simulink model "mstf_withEV"  (R2021a)
settings: Solver=VariableStepAuto  StartTime=0.0  StopTime=3  RelTol=1e-3
undefined symbols (not defined in the file or in its folder): Ion, Lithium
libraries: spsCurrentMeasurementLib x25, spsVoltageMeasurementLib x19, spsSeriesRLCBranchLib x11, spsGroundLib x6, powerlib_extras x5, dspsigops x3, spsPower3phInstantaneousLib x3, eeTotalHarmonicDistorsion x3, spsIGBTDiodeLib x2, spsUniversalBridgeLib x2, spsBatteryLib x1, spsParallelRLCBranchLib x1
settings Model: Creator=Dell  LastModifiedBy=Dell
settings SolverCC: ZeroCrossControl=DisableAll

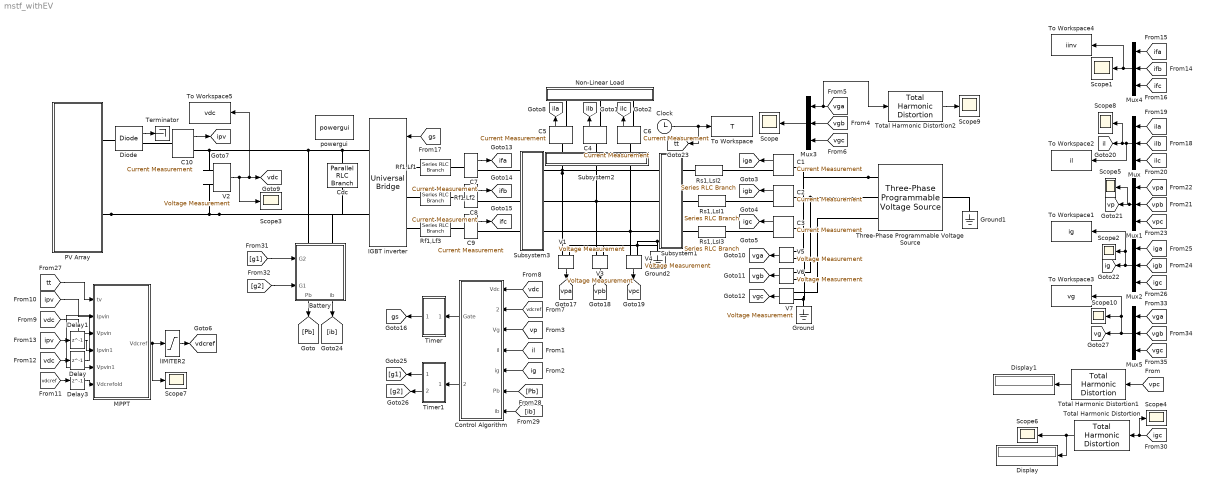
== system mstf_withEV ==
  Battery : Subsystem
      settings: PortSchema="{\"entries\":[{\"content\":{\"sides\":[{\"content\":{\"connectorIds\":[\"LConn1\",\"LConn2\"]},\"type\":\"ConnectorPlacement.EquallySpacedRectSide\",\"uuid\":\"3f024d4f-4944-46f1-a681-19b9b6f5c2e3\"},{\"content\":{\"connectorIds\":[\"Out1\",\"Out2\"],\"side\":\"RIGHT\"},\"type\":\"ConnectorPlacement.EquallySpacedRectSide\",\"uuid\":\"ba9189b8-b241-4d0f-92c2-ffae32477602\"},{\"content\":{\"connectorIds\":[\"In1\",\"In2\"],\"side\":\"TOP\"},\"type\":\"ConnectorPlacement.EquallySpacedRectSide\",\"uuid\":\"2b5a68b6-4f88-4313-be0a-70c6e84ce948\"}]},\"type\":\"ConnectorPlacement.EquallySpacedConnector\",\"uuid\":\"57f7ac83-2601-4f06-be16-46ca99d36a1f\"}],\"packageUris\":[\"http://schema.mathworks.com/mf0/Connector/R2020b\"],\"version\":\"1.0\"}"
  C{1..10} (10 alike) : spsCurrentMeasurementLib/Current Measurement  PhasorSimulation=off  OutputType=Complex  PSBequivalent=0
  Cdc : spsParallelRLCBranchLib/Parallel RLC Branch  LConnTagsString=a  RConnTagsString=__new0  BranchType=C  Resistance=10  Inductance=1.0  SetiL0=off  InitialCurrent=0  Capacitance=800e-6  Setx0=on  InitialVoltage=810  Measurements=None
  Clock : Clock
  Control Algorithm : Subsystem
  Delay : Delay  DelayLength=1  InitialCondition=0  InputProcessing=Columns as channels (frame based)
  Delay1 : Delay  DelayLength=1  InitialCondition=0  InputProcessing=Columns as channels (frame based)
  Delay3 : Delay  DelayLength=1  InitialCondition=810  InputProcessing=Columns as channels (frame based)
  Diode : spsDiodeLib/Diode  Ron=0.001  Lon=0  Vf=0.8  IC=0  UseSnubber=off  Rs=500  Cs=250e-9  Measurements=on
  Display : Display
  Display1 : Display
  Ground : spsGroundLib/Ground  LConnTagsString=a
  Ground1 : spsGroundLib/Ground  LConnTagsString=a
  Ground2 : spsGroundLib/Ground  LConnTagsString=a
  IGBT inverter : spsUniversalBridgeLib/Universal Bridge  Arms=3  SnubberResistance=1e5  SnubberCapacitance=inf  Device=IGBT / Diodes  Ron=1e-3  Lon=0  ForwardVoltages="[  0  0  ]"  ForwardVoltage=0  GTOparameters=[ 10e-6 , 20e-6 ]  IGBTparameters=[ 1e-6 , 2e-6 ]  Measurements=Device voltages  Measurements_2=None  converterType=Rectifier
  MPPT : MATLAB Function  TreatAsAtomicUnit=on
  Mux{,1..5} (6 alike) : Mux  Inputs=3
  Non-Linear Load : Subsystem
  PV Array : Subsystem
  Rf1,Lf1 : spsSeriesRLCBranchLib/Series RLC Branch  LConnTagsString=__new0  RConnTagsString=__new0  BranchType=RL  Resistance=.01  Inductance=10e-3  SetiL0=off  InitialCurrent=0  Capacitance=1e-6  Setx0=off  InitialVoltage=0  Measurements=None
  Rf1,Lf2 : spsSeriesRLCBranchLib/Series RLC Branch  LConnTagsString=__new0  RConnTagsString=__new0  BranchType=RL  Resistance=.01  Inductance=10e-3  SetiL0=off  InitialCurrent=0  Capacitance=1e-6  Setx0=off  InitialVoltage=0  Measurements=None
  Rf1,Lf3 : spsSeriesRLCBranchLib/Series RLC Branch  LConnTagsString=__new0  RConnTagsString=__new0  BranchType=RL  Resistance=.01  Inductance=10e-3  SetiL0=off  InitialCurrent=0  Capacitance=1e-6  Setx0=off  InitialVoltage=0  Measurements=None
  Rs1,LsI1 : spsSeriesRLCBranchLib/Series RLC Branch  LConnTagsString=__new0  RConnTagsString=__new0  BranchType=RL  Resistance=.1  Inductance=0.5e-3  SetiL0=off  InitialCurrent=0  Capacitance=1e-6  Setx0=off  InitialVoltage=0  Measurements=None
  Rs1,LsI2 : spsSeriesRLCBranchLib/Series RLC Branch  LConnTagsString=__new0  RConnTagsString=__new0  BranchType=RL  Resistance=.1  Inductance=0.5e-3  SetiL0=off  InitialCurrent=0  Capacitance=1e-6  Setx0=off  InitialVoltage=0  Measurements=None
  Rs1,LsI3 : spsSeriesRLCBranchLib/Series RLC Branch  LConnTagsString=__new0  RConnTagsString=__new0  BranchType=RL  Resistance=.1  Inductance=0.5e-3  SetiL0=off  InitialCurrent=0  Capacitance=1e-6  Setx0=off  InitialVoltage=0  Measurements=None
  Scope{,1..10} (11 alike) : Scope
  Subsystem1 : Subsystem
  Subsystem2 : Subsystem
  Subsystem3 : Subsystem
  Terminator : Terminator
  Three-Phase Programmable Voltage Source : spsThreePhaseProgrammableVoltageSourceLib/Three-Phase Programmable Voltage Source  PositiveSequence="[400  0 50]"  VariationEntity=None  VariationType=Table of time-amplitude pairs  VariationTypeAlt=Step  VariationStep=0.5  VariationRate=10  VariationMagnitude=0.3  VariationFrequency=2  VariationTiming=[1 2]  VariationPhaseA=off  Amplitudes=[1 0.8 1.2 1.0]  TimeValues=[0 0.1 0.15 0.2]  HarmonicGeneration=on  HarmonicA=[3 0.02 -25 0]  HarmonicB=[5 0.03 35 2]  Timing="[0.05  3]"  BusType=swing  Pref=0  Qref=0  Qmin=-inf  Qmax=inf
  Timer : Subsystem
  Timer1 : Subsystem
  To Workspace : ToWorkspace  VariableName=T  SampleTime=-1
      settings: MaxDataPoints=614863
  To Workspace1 : ToWorkspace  VariableName=ig  SampleTime=-1
      settings: MaxDataPoints=614863
  To Workspace2 : ToWorkspace  VariableName=il  SampleTime=-1
      settings: MaxDataPoints=614863
  To Workspace3 : ToWorkspace  VariableName=vg  SampleTime=-1
      settings: MaxDataPoints=614863
  To Workspace4 : ToWorkspace  VariableName=iinv  SampleTime=-1
      settings: MaxDataPoints=614863
  To Workspace5 : ToWorkspace  VariableName=vdc  SampleTime=-1
      settings: MaxDataPoints=614863
  Total Harmonic Distortion : eeTotalHarmonicDistorsion/Total Harmonic Distortion  f=50  Ts=-1
      settings: SourceProductBaseCode=PS
  Total Harmonic Distortion1 : eeTotalHarmonicDistorsion/Total Harmonic Distortion  f=50  Ts=-1
      settings: SourceProductBaseCode=PS
  Total Harmonic Distortion2 : eeTotalHarmonicDistorsion/Total Harmonic Distortion  f=50  Ts=-1
      settings: SourceProductBaseCode=PS
  V{1..7} (7 alike) : spsVoltageMeasurementLib/Voltage Measurement  PhasorSimulation=off  OutputType=Complex  PSBequivalent=0
  lIMITER2 : Saturate  UpperLimit=820  LowerLimit=630
  powergui : spspowerguiLib/powergui  Priority=1  SimulationMode=Discrete  SampleTime=5e-6  frequency=60  Iterations=50  frequencyindice=50  Pbase=100e6  ErrMax=1e-4  UnitsV=kV  UnitsW=MW  buscounter=0  FunctionMessages=off  echomessages=off  EnableUseOfTLC=off  CurrentSourceSwitches=off  DisableSnubberDevices=off  DisableRonSwitches=off  DisableVfSwitches=off  DisplayEquations=off  AutomaticDiscreteSolvers=off  SolverType=Tustin  Interpol=off  ExternalGateDelay=off  methode=off  Ts=0  x0status=blocks  SPID=off  SwTol=0  HookPort=off  NonlinearTolerance=1e-4  nMaxIteration=100  ContinueOnMaxIteration=off  RestoreLinks=warning  ResistiveCurrentMeasurement=off  Frange=[0:2:500]  Ylog=off  Xlog=on  ShowGrid=off  save=off  variable=ZData  structure=sourcect6  ZoomFFT=off  StartTime=1.81  cycles=3  DisplayStyle=3  fundamental=50  FreqAxis=on  MaxFrequency=1000  frequencyindicesteady=1  RmsSteady=1  display=off
  tag scope: gs=global, ifa=global, ifb=global, ifc=global, ig=global, iga=global, igb=global, igc=global, il=global, ila=global, ilb=global, ilc=global, ipv=global, tt=global, vdc=global, vdcref=global, vg=global, vga=global, vgb=global, vgc=global, vp=global, vpa=global, vpb=global, vpc=global
  wires:
  C3/1 -> [igc]
  [iga] -> Mux2/1
  Mux5/1 -> Scope10/1, To Workspace3/1, [vg]
  [vgb] -> Mux5/2
  Battery/2(ib) -> [ib]
  V6/1 -> [vgb]
  lIMITER2/1 -> [vdcref]
  [vga] -> Mux5/1
  [ib] -> Control Algorithm/7(ib)
  Control Algorithm/2(gate2) -> Timer1/1(In1)
  Diode/1 -> Terminator/1
  [vdcref] -> Control Algorithm/2(Vdcref)
  [vgc] -> Mux5/3
  [Pb] -> Control Algorithm/6(Pb)
  [vga] -> Total Harmonic Distortion2/1, Mux3/1
  [igc] -> Scope4/1, Total Harmonic Distortion/1
  [vgc] -> Mux3/3
  Total Harmonic Distortion2/1 -> Scope9/1
  [ila] -> Mux/1
  [g1] -> Battery/1(G2)
  Battery/1(Pb) -> [Pb]
  [ig] -> Control Algorithm/5(ig)
  Mux1/1 -> Scope5/1, [vp]
  [vpc] -> Total Harmonic Distortion1/1
  [tt] -> MPPT/1(tv)
  Mux4/1 -> To Workspace4/1, Scope1/1
  Total Harmonic Distortion1/1 -> Display1/1
  [ifb] -> Mux4/2
  [vpc] -> Mux1/3
  V1/1 -> [vpa]
  Total Harmonic Distortion/1 -> Scope6/1, Display/1
  [vp] -> Control Algorithm/3(Vg)
  [igc] -> Mux2/3
  MPPT/1(Vdcref) -> Scope7/1, lIMITER2/1
  Mux3/1 -> Scope/1
  [vdcref] -> Delay3/1
  [ifc] -> Mux4/3
  [il] -> Control Algorithm/4(il)
  Mux2/1 -> To Workspace1/1, Scope2/1, [ig]
  V3/1 -> [vpb]
  V5/1 -> [vga]
  [igb] -> Mux2/2
  [vpb] -> Mux1/2
  Control Algorithm/1(Gate) -> Timer/1(In1)
  C5/1 -> [ila]
  V2/1 -> To Workspace5/1, [vdc], Scope3/1
  [vpa] -> Mux1/1
  Delay1/1 -> MPPT/4(Ipvin1)
  [ilb] -> Mux/2
  C2/1 -> [igb]
  [gs] -> IGBT inverter/1
  C4/1 -> [ilb]
  [g2] -> Battery/2(G1)
  C9/1 -> [ifc]
  Timer/1(Out1) -> [gs]
  C8/1 -> [ifb]
  Timer1/1(g1) -> [g1]
  Delay3/1 -> MPPT/6(Vdcrefold)
  C7/1 -> [ifa]
  V7/1 -> [vgc]
  Clock/1 -> [tt], To Workspace/1
  C10/1 -> [ipv]
  [ipv] -> Delay1/1
  [vdc] -> MPPT/3(Vpvin)
  Delay/1 -> MPPT/5(Vpvin1)
  C1/1 -> [iga]
  [ipv] -> MPPT/2(Ipvin)
  [ifa] -> Mux4/1
  [vdc] -> Control Algorithm/1(Vdc)
  Mux/1 -> To Workspace2/1, [il], Scope8/1
  V4/1 -> [vpc]
  Timer1/2(g2) -> [g2]
  [ilc] -> Mux/3
  C6/1 -> [ilc]
  [vgb] -> Mux3/2
  [vdc] -> Delay/1
  connections:
  V6/LConn2 -- Ground/LConn1 -- V7/LConn2 -- V5/LConn2
  V7/LConn1 -- C3/LConn1 -- Three-Phase Programmable Voltage Source/RConn3
  V2/LConn1 -- IGBT inverter/RConn1 -- Cdc/LConn1 -- Battery/LConn1 -- C10/RConn1
  Subsystem2/LConn3 -- V4/LConn1 -- Subsystem3/RConn3 -- Subsystem1/RConn3
  Subsystem1/RConn2 -- V3/LConn1 -- Subsystem2/LConn2 -- Subsystem3/RConn2
  Subsystem2/LConn1 -- Subsystem1/RConn1 -- Subsystem3/RConn1 -- V1/LConn1
  Three-Phase Programmable Voltage Source/RConn1 -- C1/LConn1 -- V5/LConn1
  Ground2/LConn1 -- V3/LConn2 -- V1/LConn2 -- V4/LConn2
  PV Array/LConn2 -- IGBT inverter/RConn2 -- Cdc/RConn1 -- Battery/LConn2 -- V2/LConn2
  Three-Phase Programmable Voltage Source/RConn2 -- C2/LConn1 -- V6/LConn1
  Rs1,LsI3/RConn1 -- C3/RConn1
  Subsystem2/RConn3 -- C6/LConn1
  C8/LConn1 -- Rf1,Lf2/RConn1
  C4/LConn1 -- Subsystem2/RConn2
  Subsystem3/LConn1 -- C7/RConn1
  IGBT inverter/LConn1 -- Rf1,Lf1/LConn1
  Diode/RConn1 -- C10/LConn1
  Rs1,LsI3/LConn1 -- Subsystem1/LConn3
  C9/LConn1 -- Rf1,Lf3/RConn1
  Non-Linear Load/LConn1 -- C5/RConn1
  C9/RConn1 -- Subsystem3/LConn3
  Non-Linear Load/LConn2 -- C4/RConn1
  C2/RConn1 -- Rs1,LsI1/RConn1
  PV Array/LConn1 -- Diode/LConn1
  Rf1,Lf2/LConn1 -- IGBT inverter/LConn2
  Rs1,LsI2/LConn1 -- Subsystem1/LConn1
  Non-Linear Load/LConn3 -- C6/RConn1
  Rs1,LsI2/RConn1 -- C1/RConn1
  Rf1,Lf3/LConn1 -- IGBT inverter/LConn3
  Ground1/LConn1 -- Three-Phase Programmable Voltage Source/LConn1
  Rf1,Lf1/RConn1 -- C7/LConn1
  C5/LConn1 -- Subsystem2/RConn1
  Rs1,LsI1/LConn1 -- Subsystem1/LConn2
  C8/RConn1 -- Subsystem3/LConn2

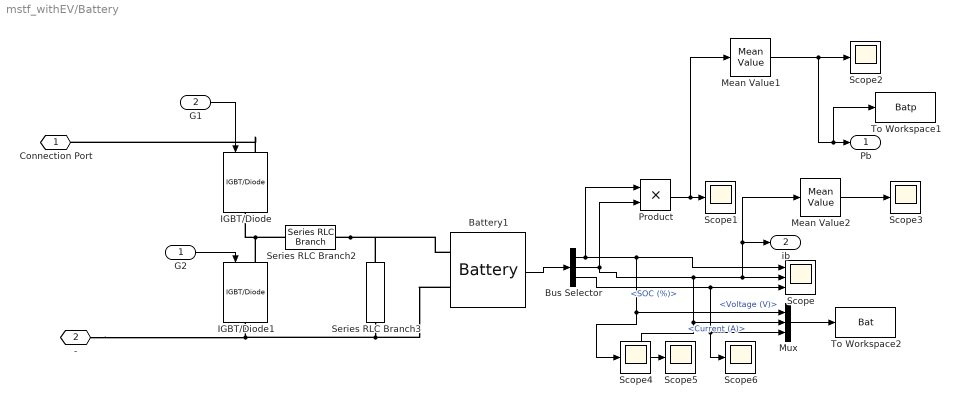
== system mstf_withEV/Battery ==
  G2 : Inport
  G1 : Inport  Port=2
  Battery1 : spsBatteryLib/Battery  BatType=Lithium-Ion  ShowTempParam=off  ThermalPreset=no  ShowAgeParam=off  NomV=300  NomQ=10  SOC=9  Batt_Tr=1  PresetModel=on  MaxQ=10  MinV=225  FullV=349.1961  Dis_rate=4.3478  R=0.3  Normal_OP=9.0435  expZone="[324.1158     0.4913043]"  current=[6.5 13 32.5]  Units=Time  Tci=20  NomT=20  T2=-30  MaxQ2=4.8  FullV2=7.1  Normal_OP2=5.655  expZone2="[6.58           1]"  Rca=0.6  ti=2000  Dp=0  Neq0=0  Tsim=1e6  Ta1=25  Qeol=5.4*0.9  Reol=0.013333*1.2  Char_age=[2.3478, 3]  Dis_age=[2.3478, 10]  N1=1500  N2=10500  N3=1000  N4=1400  Ta2=45  N5=950
  Bus Selector : BusSelector  OutputSignals=Voltage (V),Current (A),SOC (%)
  IGBT/Diode : spsIGBTDiodeLib/IGBT//Diode  Ron=1e-3  Rs=1e5  Cs=inf  Measurements=off
  IGBT/Diode1 : spsIGBTDiodeLib/IGBT//Diode  Ron=1e-3  Rs=1e5  Cs=inf  Measurements=off
  Mean Value1 : powerlib_extras/Measurements/Mean Value  Period=1/100
      settings: SourceProductBaseCode=PS
  Mean Value2 : powerlib_extras/Measurements/Mean Value  Period=1/100
      settings: SourceProductBaseCode=PS
  Mux : Mux  Inputs=3
  Product : Product
  Scope : Scope  NumInputPorts=3
  Scope{1..6} (6 alike) : Scope
  Series RLC Branch2 : spsSeriesRLCBranchLib/Series RLC Branch  LConnTagsString=__new0  RConnTagsString=__new0  BranchType=L  Resistance=1  Inductance=2e-3  SetiL0=off  InitialCurrent=0  Capacitance=1e-6  Setx0=off  InitialVoltage=0  Measurements=None
  Series RLC Branch3 : spsSeriesRLCBranchLib/Series RLC Branch  LConnTagsString=__new0  RConnTagsString=__new0  BranchType=C  Resistance=1  Inductance=1e-3  SetiL0=off  InitialCurrent=0  Capacitance=1000e-6  Setx0=off  InitialVoltage=0  Measurements=None
  To Workspace1 : ToWorkspace  VariableName=Batp  SampleTime=-1
      settings: MaxDataPoints=614863
  To Workspace2 : ToWorkspace  VariableName=Bat  SampleTime=-1
      settings: MaxDataPoints=614863
  Connection Port : PMIOPort  Side=Left
  - : PMIOPort  Port=2  Side=Left
  Pb : Outport
  ib : Outport  Port=2
  wires:
  Battery1/1 -> Bus Selector/1
  Bus Selector/1 -> Product/1, Scope/1, Mux/1, Scope4/1  "<Voltage (V)>"
  Bus Selector/2 -> Scope/2, ib/1, Mean Value2/1, Mux/2, Scope5/1, Product/2  "<Current (A)>"
  G1/1 -> IGBT/Diode/1
  G2/1 -> IGBT/Diode1/1
  Product/1 -> Mean Value1/1, Scope1/1
  Bus Selector/3 -> Scope/3, Mux/3, Scope6/1  "<SOC (%)>"
  Mean Value1/1 -> To Workspace1/1, Pb/1, Scope2/1
  Mean Value2/1 -> Scope3/1
  Mux/1 -> To Workspace2/1
  connections:
  Series RLC Branch2/RConn1 -- Battery1/LConn1 -- Series RLC Branch3/LConn1
  IGBT/Diode1/LConn1 -- Series RLC Branch2/LConn1 -- IGBT/Diode/RConn1
  Series RLC Branch3/RConn1 -- Battery1/LConn2 -- -/RConn1 -- IGBT/Diode1/RConn1
  IGBT/Diode/LConn1 -- Connection Port/RConn1

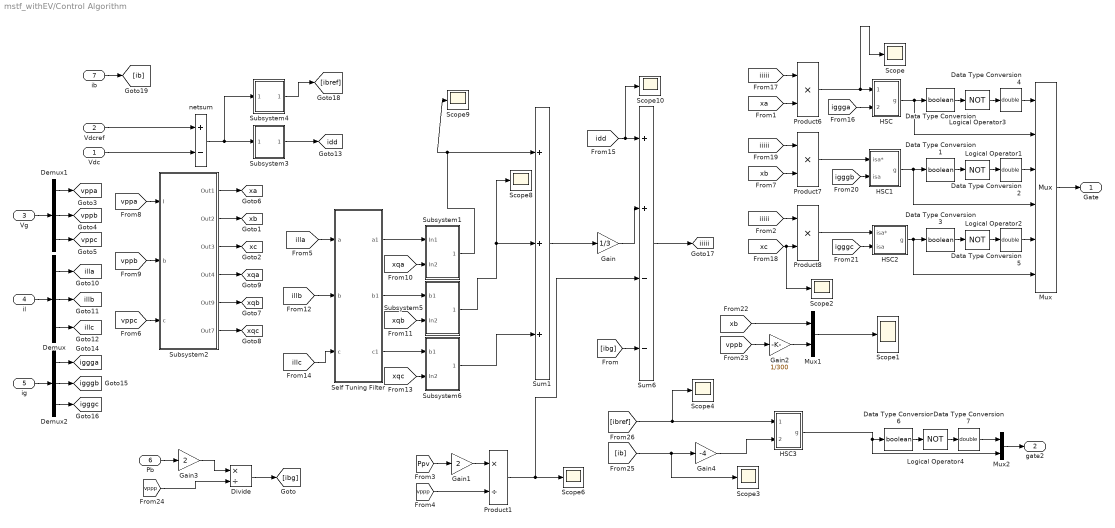
== system mstf_withEV/Control Algorithm ==
  Vdc : Inport
  Vdcref : Inport  Port=2
  Vg : Inport  Port=3
  il : Inport  Port=4
  ig : Inport  Port=5
  Pb : Inport  Port=6
  ib : Inport  Port=7
  Data Type Conversion{,1,3,6} (4 alike) : DataTypeConversion  OutDataTypeStr=boolean  SaturateOnIntegerOverflow=on  RndMeth=Zero
  Data Type Conversion{2,4..5,7} (4 alike) : DataTypeConversion  OutDataTypeStr=double  SaturateOnIntegerOverflow=on  RndMeth=Zero
  Demux : Demux  Outputs=3
  Demux1 : Demux  Outputs=3
  Demux2 : Demux  Outputs=3
  Divide : Product  Inputs=*/
  Gain : Gain  Gain=1/3
  Gain1 : Gain  Gain=2
  Gain2 : Gain  Gain=1/300
  Gain3 : Gain  Gain=2
  Gain4 : Gain  Gain=-4
  HSC : Subsystem  mask{h=.005}
      mask prompts: h "Hysteresis band (A)"
      mask help: Hysteresis Current Controller
      mask Display: plot(0,0,100,100,[45,45],[35,65],[55,55],[35,65],[45,65],[65,65],[35,55],[35,35])
  HSC1 : Subsystem  mask{h=.005}
      mask prompts: h "Hysteresis band (A)"
      mask help: Hysteresis Current Controller
      mask Display: plot(0,0,100,100,[45,45],[35,65],[55,55],[35,65],[45,65],[65,65],[35,55],[35,35])
  HSC2 : Subsystem  mask{h=.005}
      mask prompts: h "Hysteresis band (A)"
      mask help: Hysteresis Current Controller
      mask Display: plot(0,0,100,100,[45,45],[35,65],[55,55],[35,65],[45,65],[65,65],[35,55],[35,35])
  HSC3 : Subsystem  mask{h=.005}
      mask prompts: h "Hysteresis band (A)"
      mask help: Hysteresis Current Controller
      mask Display: plot(0,0,100,100,[45,45],[35,65],[55,55],[35,65],[45,65],[65,65],[35,55],[35,35])
  Logical Operator{1..4} (4 alike) : Logic  Operator=NOT  AllPortsSameDT=off  OutDataTypeStr=boolean
  Mux : Mux  Inputs=6
  Mux1 : Mux  Inputs=2
  Mux2 : Mux  Inputs=2
  Product1 : Product  Inputs=*/  RndMeth=Zero
  Product6 : Product  RndMeth=Zero
  Product7 : Product  RndMeth=Zero
  Product8 : Product  RndMeth=Zero
  Scope{,1..4,6,8..10} (9 alike) : Scope
  Self Tuning Filter : Subsystem
  Subsystem1 : Subsystem
  Subsystem2 : Subsystem
  Subsystem3 : Subsystem
  Subsystem4 : Subsystem
  Subsystem5 : Subsystem
  Subsystem6 : Subsystem
  Sum1 : Sum  Inputs=+++  InputSameDT=on  SaturateOnIntegerOverflow=on  OutDataTypeStr=Inherit: Same as first input
  Sum6 : Sum  Inputs=++--  InputSameDT=on  SaturateOnIntegerOverflow=on  OutDataTypeStr=Inherit: Same as first input
  netsum : Sum  Inputs=+-  InputSameDT=on  SaturateOnIntegerOverflow=on  OutDataTypeStr=Inherit: Same as first input
  Gate : Outport
  gate2 : Outport  Port=2
  tag scope: idd=global, iggga=global, igggb=global, igggc=global, iiiii=global, illa=global, illb=global, illc=global, vppa=global, vppb=global, vppc=global, xa=global, xb=global, xc=global, xqa=global, xqb=global, xqc=global
  wires:
  netsum/1 -> Subsystem4/1(In1), Subsystem3/1(In1)
  Subsystem2/3(Out3) -> [xc]
  Subsystem2/2(Out2) -> [xb]
  Subsystem2/1(Out1) -> [xa]
  [xa] -> Product6/2
  [xb] -> Product7/2
  [xc] -> Scope2/1, Product8/2
  HSC/1(g) -> Mux/2, Data Type Conversion/1
  Mux/1 -> Gate/1
  Product7/1 -> HSC1/1(isa*)
  Product8/1 -> HSC2/1(isa*)
  Data Type Conversion/1 -> Logical Operator3/1
  Logical Operator3/1 -> Data Type Conversion4/1
  Data Type Conversion4/1 -> Mux/1
  HSC1/1(g) -> Mux/4, Data Type Conversion1/1
  Data Type Conversion1/1 -> Logical Operator1/1
  Logical Operator1/1 -> Data Type Conversion2/1
  Data Type Conversion2/1 -> Mux/3
  Data Type Conversion3/1 -> Logical Operator2/1
  Logical Operator2/1 -> Data Type Conversion5/1
  Data Type Conversion5/1 -> Mux/5
  HSC2/1(g) -> Mux/6, Data Type Conversion3/1
  [Ppv] -> Gain1/1
  Gain1/1 -> Product1/1
  [vppp] -> Product1/2
  Product1/1 -> Sum6/3, Scope6/1
  Subsystem3/1(Out1) -> [idd]
  il/1 -> Demux/1
  Vg/1 -> Demux1/1
  ig/1 -> Demux2/1
  Demux1/1 -> [vppa]
  Demux1/2 -> [vppb]
  Demux1/3 -> [vppc]
  [vppa] -> Subsystem2/1(I)
  [vppb] -> Subsystem2/2(b)
  [vppc] -> Subsystem2/3(c)
  Subsystem2/4(Out4) -> [xqa]
  Subsystem2/5(Out9) -> [xqb]
  Subsystem2/6(Out7) -> [xqc]
  Demux/3 -> [illc]
  Demux/2 -> [illb]
  Demux/1 -> [illa]
  Subsystem1/1(Out1) -> Scope9/1, Sum1/1
  Subsystem5/1(Out1) -> Scope8/1, Sum1/2
  Subsystem6/1(Out1) -> Sum1/3
  Demux2/1 -> [iggga]
  Demux2/2 -> [igggb]
  Demux2/3 -> [igggc]
  Sum6/1 -> [iiiii]
  [iiiii] -> Product7/1
  [iiiii] -> Product6/1
  [iiiii] -> Product8/1
  [iggga] -> HSC/2(isa)
  [igggb] -> HSC1/2(isa)
  [igggc] -> HSC2/2(isa)
  [xb] -> Mux1/1
  [vppb] -> Gain2/1
  Mux1/1 -> Scope1/1
  Gain2/1 -> Mux1/2
  Vdcref/1 -> netsum/1
  Product6/1 -> Scope/1, HSC/1(isa*)
  [idd] -> Scope10/1, Sum6/1
  Vdc/1 -> netsum/2
  Sum1/1 -> Gain/1
  Gain/1 -> Sum6/2
  Pb/1 -> Gain3/1
  Gain3/1 -> Divide/1
  [vppp] -> Divide/2
  Divide/1 -> [ibg]
  [ibg] -> Sum6/4
  ib/1 -> [ib]
  [ibref] -> Scope4/1, HSC3/1(isa*)
  Logical Operator4/1 -> Data Type Conversion7/1
  Data Type Conversion6/1 -> Logical Operator4/1
  HSC3/1(g) -> Mux2/2, Data Type Conversion6/1
  Data Type Conversion7/1 -> Mux2/1
  Mux2/1 -> gate2/1
  [ib] -> Scope3/1, Gain4/1
  Gain4/1 -> HSC3/2(isa)
  Subsystem4/1(Out1) -> [ibref]
  [illb] -> Self Tuning Filter/2(b)
  Self Tuning Filter/2(b1) -> Subsystem5/1(b1)
  [illa] -> Self Tuning Filter/1(a)
  [illc] -> Self Tuning Filter/3(c)
  Self Tuning Filter/1(a1) -> Subsystem1/1(In1)
  [xqa] -> Subsystem1/2(In2)
  [xqb] -> Subsystem5/2(In2)
  Self Tuning Filter/3(c1) -> Subsystem6/1(b1)
  [xqc] -> Subsystem6/2(In2)

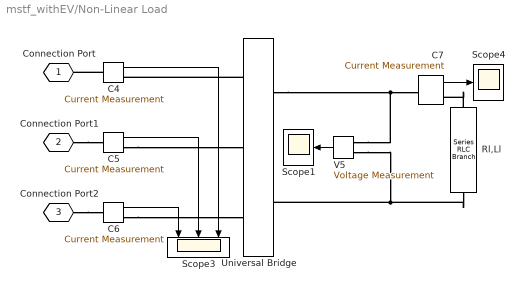
== system mstf_withEV/Non-Linear Load ==
  C{4..7} (4 alike) : spsCurrentMeasurementLib/Current Measurement  PhasorSimulation=off  OutputType=Complex  PSBequivalent=0
  Rl,Ll : spsSeriesRLCBranchLib/Series RLC Branch  LConnTagsString=__new0  RConnTagsString=__new0  BranchType=RL  Resistance=200  Inductance=25e-3  SetiL0=off  InitialCurrent=0  Capacitance=1.0  Setx0=off  InitialVoltage=0  Measurements=None
  Scope1 : Scope
  Scope3 : Scope  NumInputPorts=3
  Scope4 : Scope
  Universal Bridge : spsUniversalBridgeLib/Universal Bridge  Arms=3  SnubberResistance=500  SnubberCapacitance=.1e-6  Device=Diodes  Ron=1e-3  Lon=0  ForwardVoltages="[  0  0  ]"  ForwardVoltage=.8  GTOparameters=[ 10e-6 , 20e-6 ]  IGBTparameters=[ 1e-6 , 2e-6 ]  Measurements=Device voltages  Measurements_2=None  converterType=Rectifier
  V5 : spsVoltageMeasurementLib/Voltage Measurement  PhasorSimulation=off  OutputType=Complex  PSBequivalent=0
  Connection Port : PMIOPort  Tag=PMCPort  Side=Left
  Connection Port1 : PMIOPort  Tag=PMCPort  Port=2  Side=Left
  Connection Port2 : PMIOPort  Tag=PMCPort  Port=3  Side=Left
  wires:
  C7/1 -> Scope4/1
  V5/1 -> Scope1/1
  C6/1 -> Scope3/1
  C5/1 -> Scope3/2
  C4/1 -> Scope3/3
  connections:
  Universal Bridge/RConn1 -- V5/LConn1 -- C7/LConn1
  Rl,Ll/LConn1 -- C7/RConn1
  Rl,Ll/RConn1 -- V5/LConn2 -- Universal Bridge/RConn2
  C4/LConn1 -- Connection Port/RConn1
  Connection Port2/RConn1 -- C6/LConn1
  Connection Port1/RConn1 -- C5/LConn1
  C6/RConn1 -- Universal Bridge/LConn3
  C5/RConn1 -- Universal Bridge/LConn2
  Universal Bridge/LConn1 -- C4/RConn1

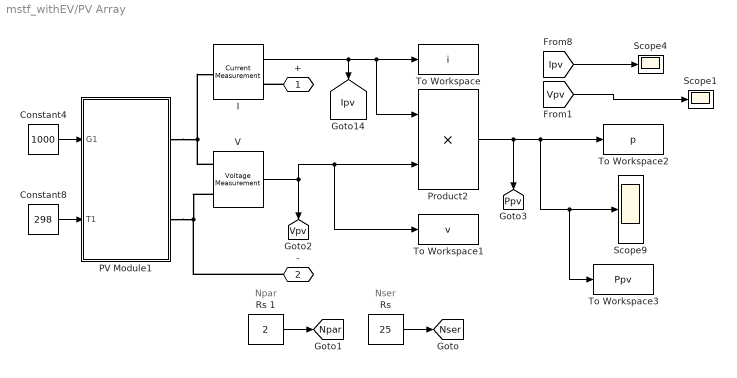
== system mstf_withEV/PV Array ==
  note: Nser
  note: Npar
  Constant4 : Constant  Value=1000
  Constant8 : Constant  Value=298
  I : spsCurrentMeasurementLib/Current Measurement  PhasorSimulation=off  OutputType=Complex  PSBequivalent=0
  PV Module1 : Subsystem
  Product2 : Product  RndMeth=Zero
  "Rs " : Constant  Value=25
  Rs 1 : Constant  Value=2
  Scope1 : Scope
  Scope4 : Scope
  Scope9 : Scope
  To Workspace : ToWorkspace  VariableName=i  SaveFormat=Timeseries  SampleTime=-1
  To Workspace1 : ToWorkspace  VariableName=v  SaveFormat=Timeseries  SampleTime=-1
  To Workspace2 : ToWorkspace  VariableName=p  SampleTime=-1
  To Workspace3 : ToWorkspace  VariableName=Ppv  SampleTime=-1
      settings: MaxDataPoints=614863
  "V " : spsVoltageMeasurementLib/Voltage Measurement  PhasorSimulation=off  OutputType=Complex  PSBequivalent=0
  + : PMIOPort  Side=Left
  - : PMIOPort  Port=2  Side=Left
  tag scope: Ipv=global, Npar=global, Nser=global, Ppv=global, Vpv=global
  wires:
  Constant4/1 -> PV Module1/1(G1)
  Constant8/1 -> PV Module1/2(T1)
  "Rs "/1 -> [Nser]
  Rs 1/1 -> [Npar]
  Product2/1 -> To Workspace2/1, To Workspace3/1, Scope9/1, [Ppv]
  I/1 -> Product2/1, To Workspace/1, [Ipv]
  "V "/1 -> [Vpv], To Workspace1/1, Product2/2
  [Ipv] -> Scope4/1
  [Vpv] -> Scope1/1
  connections:
  "V "/LConn2 -- -/RConn1 -- PV Module1/RConn2
  "V "/LConn1 -- I/LConn1 -- PV Module1/RConn1
  +/RConn1 -- I/RConn1

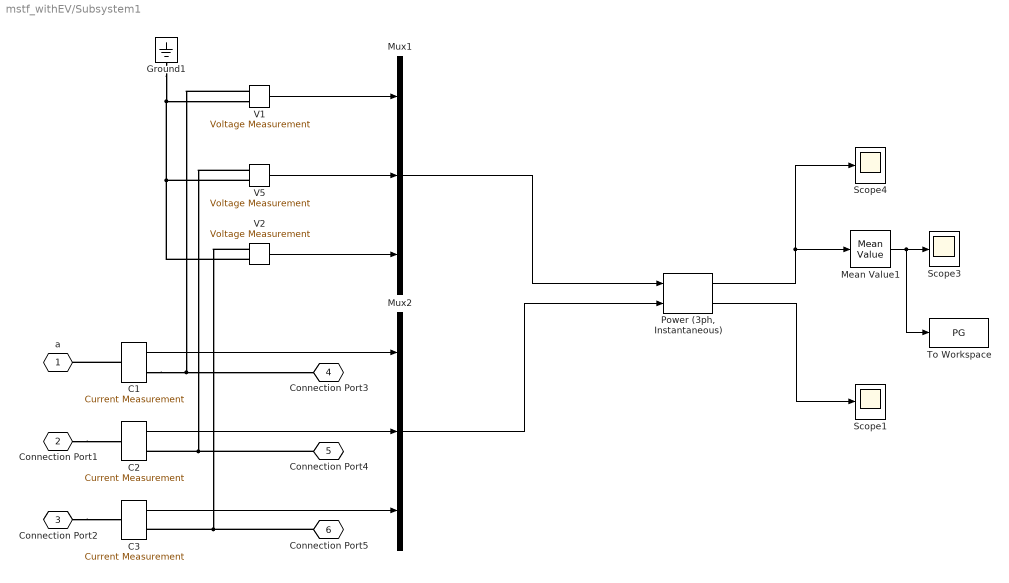
== system mstf_withEV/Subsystem1 ==
  C1 : spsCurrentMeasurementLib/Current Measurement  PhasorSimulation=off  OutputType=Complex  PSBequivalent=0
  C2 : spsCurrentMeasurementLib/Current Measurement  PhasorSimulation=off  OutputType=Complex  PSBequivalent=0
  C3 : spsCurrentMeasurementLib/Current Measurement  PhasorSimulation=off  OutputType=Complex  PSBequivalent=0
  Ground1 : spsGroundLib/Ground  LConnTagsString=a
  Mean Value1 : powerlib_extras/Measurements/Mean Value  Period=1/100
      settings: SourceProductBaseCode=PS
  Mux1 : Mux  Inputs=3
  Mux2 : Mux  Inputs=3
  "Power (3ph, Instantaneous)" : spsPower3phInstantaneousLib/Power (3ph, Instantaneous)
  Scope1 : Scope
  Scope3 : Scope
  Scope4 : Scope
  To Workspace : ToWorkspace  VariableName=PG  SampleTime=-1
      settings: MaxDataPoints=614863
  V1 : spsVoltageMeasurementLib/Voltage Measurement  PhasorSimulation=off  OutputType=Complex  PSBequivalent=0
  V2 : spsVoltageMeasurementLib/Voltage Measurement  PhasorSimulation=off  OutputType=Complex  PSBequivalent=0
  V5 : spsVoltageMeasurementLib/Voltage Measurement  PhasorSimulation=off  OutputType=Complex  PSBequivalent=0
  a : PMIOPort  Tag=PMCPort  Side=Left
  Connection Port1 : PMIOPort  Tag=PMCPort  Port=2  Side=Left
  Connection Port2 : PMIOPort  Tag=PMCPort  Port=3  Side=Left
  Connection Port3 : PMIOPort  Tag=PMCPort  Port=4  Side=Right
  Connection Port4 : PMIOPort  Tag=PMCPort  Port=5  Side=Right
  Connection Port5 : PMIOPort  Tag=PMCPort  Port=6  Side=Right
  wires:
  Mean Value1/1 -> To Workspace/1, Scope3/1
  C1/1 -> Mux2/1
  C2/1 -> Mux2/2
  C3/1 -> Mux2/3
  V1/1 -> Mux1/1
  V5/1 -> Mux1/2
  V2/1 -> Mux1/3
  Mux1/1 -> "Power (3ph, Instantaneous)"/1
  Mux2/1 -> "Power (3ph, Instantaneous)"/2
  "Power (3ph, Instantaneous)"/2 -> Scope1/1
  "Power (3ph, Instantaneous)"/1 -> Scope4/1, Mean Value1/1
  connections:
  C1/LConn1 -- a/RConn1
  C3/RConn1 -- Connection Port5/RConn1 -- V2/LConn1
  C2/RConn1 -- Connection Port4/RConn1 -- V5/LConn1
  V1/LConn1 -- C1/RConn1 -- Connection Port3/RConn1
  Ground1/LConn1 -- V1/LConn2 -- V2/LConn2 -- V5/LConn2
  Connection Port2/RConn1 -- C3/LConn1
  Connection Port1/RConn1 -- C2/LConn1

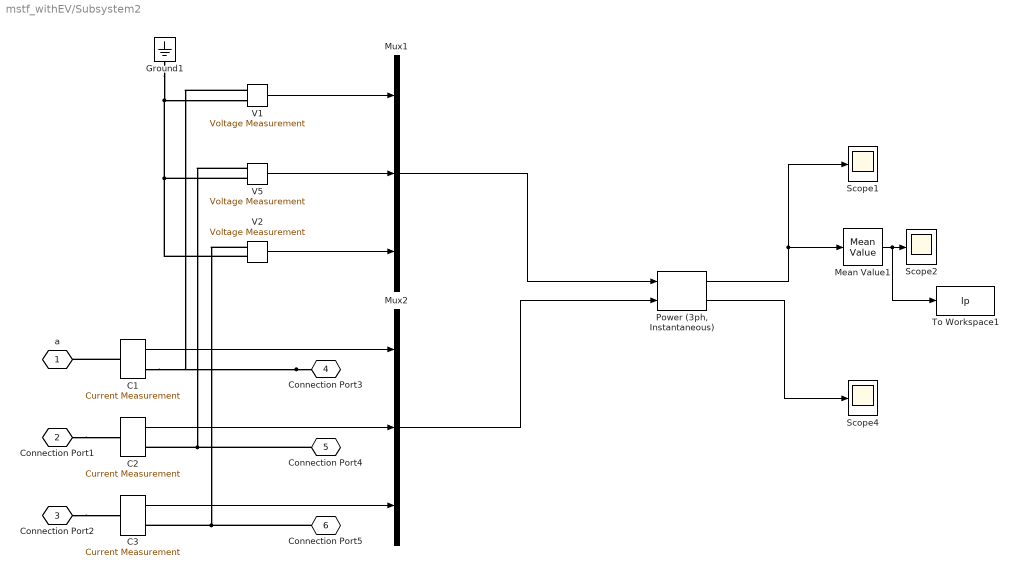
== system mstf_withEV/Subsystem2 ==
  C1 : spsCurrentMeasurementLib/Current Measurement  PhasorSimulation=off  OutputType=Complex  PSBequivalent=0
  C2 : spsCurrentMeasurementLib/Current Measurement  PhasorSimulation=off  OutputType=Complex  PSBequivalent=0
  C3 : spsCurrentMeasurementLib/Current Measurement  PhasorSimulation=off  OutputType=Complex  PSBequivalent=0
  Ground1 : spsGroundLib/Ground  LConnTagsString=a
  Mean Value1 : powerlib_extras/Measurements/Mean Value  Period=1/100
      settings: SourceProductBaseCode=PS
  Mux1 : Mux  Inputs=3
  Mux2 : Mux  Inputs=3
  "Power (3ph, Instantaneous)" : spsPower3phInstantaneousLib/Power (3ph, Instantaneous)
  Scope1 : Scope
  Scope2 : Scope
  Scope4 : Scope
  To Workspace1 : ToWorkspace  VariableName=lp  SampleTime=-1
      settings: MaxDataPoints=614863
  V1 : spsVoltageMeasurementLib/Voltage Measurement  PhasorSimulation=off  OutputType=Complex  PSBequivalent=0
  V2 : spsVoltageMeasurementLib/Voltage Measurement  PhasorSimulation=off  OutputType=Complex  PSBequivalent=0
  V5 : spsVoltageMeasurementLib/Voltage Measurement  PhasorSimulation=off  OutputType=Complex  PSBequivalent=0
  a : PMIOPort  Tag=PMCPort  Side=Left
  Connection Port1 : PMIOPort  Tag=PMCPort  Port=2  Side=Left
  Connection Port2 : PMIOPort  Tag=PMCPort  Port=3  Side=Left
  Connection Port3 : PMIOPort  Tag=PMCPort  Port=4  Side=Right
  Connection Port4 : PMIOPort  Tag=PMCPort  Port=5  Side=Right
  Connection Port5 : PMIOPort  Tag=PMCPort  Port=6  Side=Right
  wires:
  "Power (3ph, Instantaneous)"/1 -> Scope1/1, Mean Value1/1
  "Power (3ph, Instantaneous)"/2 -> Scope4/1
  Mux2/1 -> "Power (3ph, Instantaneous)"/2
  Mux1/1 -> "Power (3ph, Instantaneous)"/1
  V2/1 -> Mux1/3
  V5/1 -> Mux1/2
  V1/1 -> Mux1/1
  C3/1 -> Mux2/3
  C2/1 -> Mux2/2
  C1/1 -> Mux2/1
  Mean Value1/1 -> To Workspace1/1, Scope2/1
  connections:
  Connection Port1/RConn1 -- C2/LConn1
  Connection Port2/RConn1 -- C3/LConn1
  V5/LConn2 -- V2/LConn2 -- V1/LConn2 -- Ground1/LConn1
  Connection Port3/RConn1 -- C1/RConn1 -- V1/LConn1
  V5/LConn1 -- Connection Port4/RConn1 -- C2/RConn1
  V2/LConn1 -- Connection Port5/RConn1 -- C3/RConn1
  C1/LConn1 -- a/RConn1

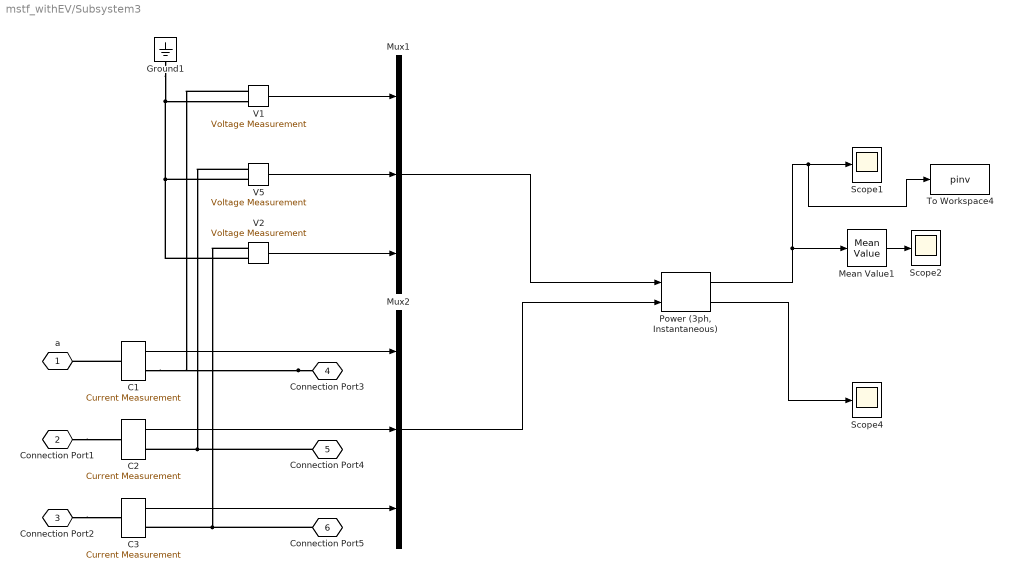
== system mstf_withEV/Subsystem3 ==
  C1 : spsCurrentMeasurementLib/Current Measurement  PhasorSimulation=off  OutputType=Complex  PSBequivalent=0
  C2 : spsCurrentMeasurementLib/Current Measurement  PhasorSimulation=off  OutputType=Complex  PSBequivalent=0
  C3 : spsCurrentMeasurementLib/Current Measurement  PhasorSimulation=off  OutputType=Complex  PSBequivalent=0
  Ground1 : spsGroundLib/Ground  LConnTagsString=a
  Mean Value1 : powerlib_extras/Measurements/Mean Value  Period=1/100
      settings: SourceProductBaseCode=PS
  Mux1 : Mux  Inputs=3
  Mux2 : Mux  Inputs=3
  "Power (3ph, Instantaneous)" : spsPower3phInstantaneousLib/Power (3ph, Instantaneous)
  Scope1 : Scope
  Scope2 : Scope
  Scope4 : Scope
  To Workspace4 : ToWorkspace  VariableName=pinv  SampleTime=-1
      settings: MaxDataPoints=614863
  V1 : spsVoltageMeasurementLib/Voltage Measurement  PhasorSimulation=off  OutputType=Complex  PSBequivalent=0
  V2 : spsVoltageMeasurementLib/Voltage Measurement  PhasorSimulation=off  OutputType=Complex  PSBequivalent=0
  V5 : spsVoltageMeasurementLib/Voltage Measurement  PhasorSimulation=off  OutputType=Complex  PSBequivalent=0
  a : PMIOPort  Tag=PMCPort  Side=Left
  Connection Port1 : PMIOPort  Tag=PMCPort  Port=2  Side=Left
  Connection Port2 : PMIOPort  Tag=PMCPort  Port=3  Side=Left
  Connection Port3 : PMIOPort  Tag=PMCPort  Port=4  Side=Right
  Connection Port4 : PMIOPort  Tag=PMCPort  Port=5  Side=Right
  Connection Port5 : PMIOPort  Tag=PMCPort  Port=6  Side=Right
  wires:
  "Power (3ph, Instantaneous)"/1 -> To Workspace4/1, Scope1/1, Mean Value1/1
  "Power (3ph, Instantaneous)"/2 -> Scope4/1
  Mux2/1 -> "Power (3ph, Instantaneous)"/2
  Mux1/1 -> "Power (3ph, Instantaneous)"/1
  V2/1 -> Mux1/3
  V5/1 -> Mux1/2
  V1/1 -> Mux1/1
  C3/1 -> Mux2/3
  C2/1 -> Mux2/2
  C1/1 -> Mux2/1
  Mean Value1/1 -> Scope2/1
  connections:
  Connection Port1/RConn1 -- C2/LConn1
  Connection Port2/RConn1 -- C3/LConn1
  V5/LConn2 -- V2/LConn2 -- V1/LConn2 -- Ground1/LConn1
  Connection Port3/RConn1 -- C1/RConn1 -- V1/LConn1
  V5/LConn1 -- Connection Port4/RConn1 -- C2/RConn1
  V2/LConn1 -- Connection Port5/RConn1 -- C3/RConn1
  C1/LConn1 -- a/RConn1

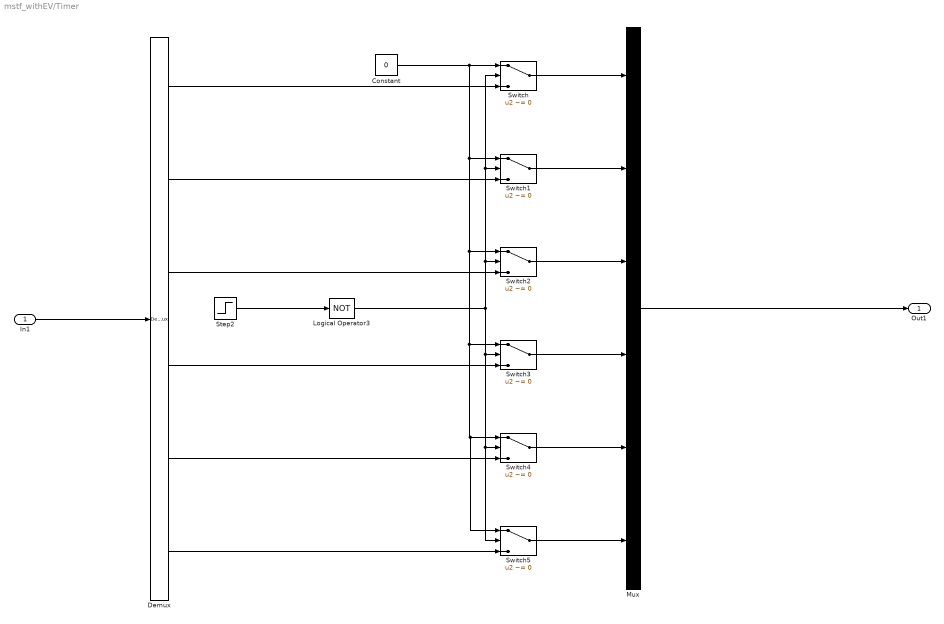
== system mstf_withEV/Timer ==
  In1 : Inport
  Constant : Constant  Value=0
  Demux : Demux  Outputs=6
  Logical Operator3 : Logic  Operator=NOT  AllPortsSameDT=off  OutDataTypeStr=boolean
  Mux : Mux  Inputs=6
  Step2 : Step  Time=.6  SampleTime=0
  Switch{,1..5} (6 alike) : Switch  Criteria=u2 ~= 0
  Out1 : Outport
  wires:
  In1/1 -> Demux/1
  Constant/1 -> Switch1/1, Switch2/1, Switch5/1, Switch4/1, Switch3/1, Switch/1
  Demux/6 -> Switch5/3
  Demux/5 -> Switch4/3
  Demux/4 -> Switch3/3
  Demux/3 -> Switch2/3
  Demux/2 -> Switch1/3
  Demux/1 -> Switch/3
  Step2/1 -> Logical Operator3/1
  Switch/1 -> Mux/1
  Switch1/1 -> Mux/2
  Switch2/1 -> Mux/3
  Switch3/1 -> Mux/4
  Switch4/1 -> Mux/5
  Switch5/1 -> Mux/6
  Mux/1 -> Out1/1
  Logical Operator3/1 -> Switch3/2, Switch5/2, Switch4/2, Switch/2, Switch1/2, Switch2/2

== system mstf_withEV/Timer1 ==
  In1 : Inport
  Constant : Constant  Value=0
  Demux : Demux  Outputs=2
  Logical Operator3 : Logic  Operator=NOT  AllPortsSameDT=off  OutDataTypeStr=boolean
  Step2 : Step  Time=.6  SampleTime=0
  Switch2 : Switch  Criteria=u2 ~= 0
  Switch3 : Switch  Criteria=u2 ~= 0
  g1 : Outport
  g2 : Outport  Port=2
  wires:
  Constant/1 -> Switch3/1, Switch2/1
  Step2/1 -> Logical Operator3/1
  Logical Operator3/1 -> Switch3/2, Switch2/2
  In1/1 -> Demux/1
  Demux/1 -> Switch2/3
  Demux/2 -> Switch3/3
  Switch2/1 -> g1/1
  Switch3/1 -> g2/1

== system mstf_withEV/Control Algorithm/HSC ==
  isa* : Inport
  isa : Inport  Port=2
  Relay : Relay  OnSwitchValue=h/2  OffSwitchValue=-h/2
  Sum1 : Sum  Inputs=-+  InputSameDT=on  SaturateOnIntegerOverflow=on  OutDataTypeStr=Inherit: Same as first input
  g : Outport  InitialOutput=0
  wires:
  Sum1/1 -> Relay/1
  Relay/1 -> g/1
  isa/1 -> Sum1/1
  isa*/1 -> Sum1/2

== system mstf_withEV/Control Algorithm/HSC1 ==
  isa* : Inport
  isa : Inport  Port=2
  Relay : Relay  OnSwitchValue=h/2  OffSwitchValue=-h/2
  Sum1 : Sum  Inputs=-+  InputSameDT=on  SaturateOnIntegerOverflow=on  OutDataTypeStr=Inherit: Same as first input
  g : Outport  InitialOutput=0
  wires:
  isa*/1 -> Sum1/2
  isa/1 -> Sum1/1
  Relay/1 -> g/1
  Sum1/1 -> Relay/1

== system mstf_withEV/Control Algorithm/HSC2 ==
  isa* : Inport
  isa : Inport  Port=2
  Relay : Relay  OnSwitchValue=h/2  OffSwitchValue=-h/2
  Sum1 : Sum  Inputs=-+  InputSameDT=on  SaturateOnIntegerOverflow=on  OutDataTypeStr=Inherit: Same as first input
  g : Outport  InitialOutput=0
  wires:
  Sum1/1 -> Relay/1
  Relay/1 -> g/1
  isa/1 -> Sum1/1
  isa*/1 -> Sum1/2

== system mstf_withEV/Control Algorithm/HSC3 ==
  isa* : Inport
  isa : Inport  Port=2
  Relay : Relay  OnSwitchValue=h/2  OffSwitchValue=-h/2
  Sum1 : Sum  Inputs=-+  InputSameDT=on  SaturateOnIntegerOverflow=on  OutDataTypeStr=Inherit: Same as first input
  g : Outport  InitialOutput=0
  wires:
  Sum1/1 -> Relay/1
  Relay/1 -> g/1
  isa/1 -> Sum1/1
  isa*/1 -> Sum1/2

== system mstf_withEV/Control Algorithm/Self Tuning Filter ==
  a : Inport
  b : Inport  Port=2
  c : Inport  Port=3
  Subsystem2 : Subsystem
  a1 : Outport
  b1 : Outport  Port=2
  c1 : Outport  Port=3
  wires:
  a/1 -> Subsystem2/1(a)
  Subsystem2/1(a1) -> a1/1
  b/1 -> Subsystem2/2(a2)
  c/1 -> Subsystem2/3(a4)
  Subsystem2/2(a3) -> b1/1
  Subsystem2/3(a5) -> c1/1

== system mstf_withEV/Control Algorithm/Subsystem1 ==
  In1 : Inport
  In2 : Inport  Port=2
  Abs : Abs
  Constant5 : Constant  Value=0  VectorParams1D=off
  Data Type Conversion1 : DataTypeConversion  OutDataTypeStr=double  SaturateOnIntegerOverflow=on  RndMeth=Zero
  Relational Operator2 : RelationalOperator  RndMeth=Nearest  InputSameDT=on
  Sample and Hold : dspsigops/Sample and Hold  trig=Either edge  initCond=0  latchinput=off
  Out1 : Outport
  wires:
  In1/1 -> Sample and Hold/1
  Constant5/1 -> Relational Operator2/2
  Relational Operator2/1 -> Data Type Conversion1/1
  In2/1 -> Relational Operator2/1
  Data Type Conversion1/1 -> Sample and Hold/Trigger
  Sample and Hold/1 -> Abs/1
  Abs/1 -> Out1/1

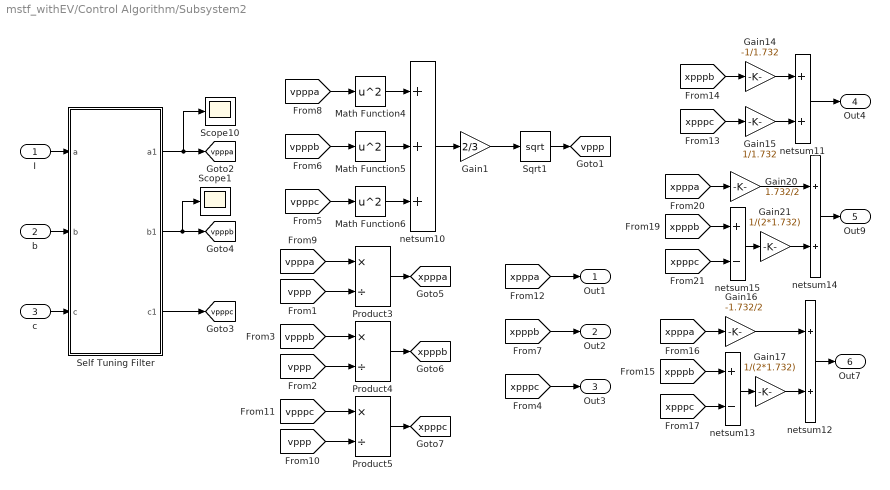
== system mstf_withEV/Control Algorithm/Subsystem2 ==
  I : Inport
  b : Inport  Port=2
  c : Inport  Port=3
  Gain1 : Gain  Gain=2/3
  Gain14 : Gain  Gain=-1/1.732
  Gain15 : Gain  Gain=1/1.732
  Gain16 : Gain  Gain=-1.732/2
  Gain17 : Gain  Gain=1/(2*1.732)
  Gain20 : Gain  Gain=1.732/2
  Gain21 : Gain  Gain=1/(2*1.732)
  Math Function4 : Math  Operator=square  SignedPower=on  SaturateOnIntegerOverflow=on
  Math Function5 : Math  Operator=square  SignedPower=on  SaturateOnIntegerOverflow=on
  Math Function6 : Math  Operator=square  SignedPower=on  SaturateOnIntegerOverflow=on
  Product3 : Product  Inputs=*/  RndMeth=Zero
  Product4 : Product  Inputs=*/  RndMeth=Zero
  Product5 : Product  Inputs=*/  RndMeth=Zero
  Scope1 : Scope
  Scope10 : Scope
  Self Tuning Filter : Subsystem
  Sqrt1 : Sqrt  SaturateOnIntegerOverflow=on
  netsum10 : Sum  Inputs=+++  InputSameDT=on  SaturateOnIntegerOverflow=on  OutDataTypeStr=Inherit: Same as first input
  netsum11 : Sum  InputSameDT=on  SaturateOnIntegerOverflow=on  OutDataTypeStr=Inherit: Same as first input
  netsum12 : Sum  InputSameDT=on  SaturateOnIntegerOverflow=on  OutDataTypeStr=Inherit: Same as first input
  netsum13 : Sum  Inputs=+-  InputSameDT=on  SaturateOnIntegerOverflow=on  OutDataTypeStr=Inherit: Same as first input
  netsum14 : Sum  InputSameDT=on  SaturateOnIntegerOverflow=on  OutDataTypeStr=Inherit: Same as first input
  netsum15 : Sum  Inputs=+-  InputSameDT=on  SaturateOnIntegerOverflow=on  OutDataTypeStr=Inherit: Same as first input
  Out1 : Outport
  Out2 : Outport  Port=2
  Out3 : Outport  Port=3
  Out4 : Outport  Port=4
  Out9 : Outport  Port=5
  Out7 : Outport  Port=6
  tag scope: vppp=global, vpppa=global, vpppb=global, vpppc=global, xpppa=global, xpppb=global, xpppc=global
  wires:
  Math Function4/1 -> netsum10/1
  Math Function5/1 -> netsum10/2
  Math Function6/1 -> netsum10/3
  netsum10/1 -> Gain1/1
  Sqrt1/1 -> [vppp]
  I/1 -> Self Tuning Filter/1(a)
  c/1 -> Self Tuning Filter/3(c)
  b/1 -> Self Tuning Filter/2(b)
  [vpppb] -> Math Function5/1
  [vpppa] -> Math Function4/1
  [vpppc] -> Math Function6/1
  [vpppa] -> Product3/1
  [vppp] -> Product3/2
  [vppp] -> Product4/2
  [vpppb] -> Product4/1
  [vpppc] -> Product5/1
  [vppp] -> Product5/2
  Product3/1 -> [xpppa]
  Product4/1 -> [xpppb]
  Product5/1 -> [xpppc]
  [xpppa] -> Out1/1
  [xpppb] -> Out2/1
  [xpppc] -> Out3/1
  [xpppb] -> Gain14/1
  Gain14/1 -> netsum11/1
  Gain15/1 -> netsum11/2
  [xpppc] -> Gain15/1
  netsum11/1 -> Out4/1
  netsum14/1 -> Out9/1
  [xpppb] -> netsum15/1
  Gain21/1 -> netsum14/2
  Gain20/1 -> netsum14/1
  [xpppa] -> Gain20/1
  [xpppc] -> netsum15/2
  netsum15/1 -> Gain21/1
  netsum13/1 -> Gain17/1
  [xpppc] -> netsum13/2
  [xpppa] -> Gain16/1
  Gain16/1 -> netsum12/1
  Gain17/1 -> netsum12/2
  [xpppb] -> netsum13/1
  netsum12/1 -> Out7/1
  Gain1/1 -> Sqrt1/1
  Self Tuning Filter/1(a1) -> [vpppa], Scope10/1
  Self Tuning Filter/2(b1) -> [vpppb], Scope1/1
  Self Tuning Filter/3(c1) -> [vpppc]

== system mstf_withEV/Control Algorithm/Subsystem3 ==
  In1 : Inport
  Add : Sum  Inputs=+++
  Derivative : Derivative
  Gain : Gain  Gain=0.3
  Gain1 : Gain
  Gain2 : Gain  Gain=.00001
  Integrator : Integrator  ZeroCross=off
  Out1 : Outport
  wires:
  In1/1 -> Gain2/1, Gain/1, Gain1/1
  Gain1/1 -> Integrator/1
  Gain2/1 -> Derivative/1
  Gain/1 -> Add/1
  Derivative/1 -> Add/3
  Add/1 -> Out1/1
  Integrator/1 -> Add/2

== system mstf_withEV/Control Algorithm/Subsystem4 ==
  In1 : Inport
  Add : Sum  Inputs=+++
  Derivative : Derivative
  Gain : Gain  Gain=0.3
  Gain1 : Gain  Gain=0.4
  Gain2 : Gain  Gain=.00001
  Integrator : Integrator  ZeroCross=off
  Out1 : Outport
  wires:
  In1/1 -> Gain2/1, Gain/1, Gain1/1
  Gain1/1 -> Integrator/1
  Gain2/1 -> Derivative/1
  Gain/1 -> Add/1
  Derivative/1 -> Add/3
  Add/1 -> Out1/1
  Integrator/1 -> Add/2

== system mstf_withEV/Control Algorithm/Subsystem5 ==
  b1 : Inport
  In2 : Inport  Port=2
  Abs : Abs
  Constant5 : Constant  Value=0  VectorParams1D=off
  Data Type Conversion1 : DataTypeConversion  OutDataTypeStr=double  SaturateOnIntegerOverflow=on  RndMeth=Zero
  Relational Operator2 : RelationalOperator  RndMeth=Nearest  InputSameDT=on
  Sample and Hold : dspsigops/Sample and Hold  trig=Either edge  initCond=0  latchinput=off
  Out1 : Outport
  wires:
  b1/1 -> Sample and Hold/1
  Constant5/1 -> Relational Operator2/2
  Relational Operator2/1 -> Data Type Conversion1/1
  In2/1 -> Relational Operator2/1
  Data Type Conversion1/1 -> Sample and Hold/Trigger
  Sample and Hold/1 -> Abs/1
  Abs/1 -> Out1/1

== system mstf_withEV/Control Algorithm/Subsystem6 ==
  b1 : Inport
  In2 : Inport  Port=2
  Abs : Abs
  Constant5 : Constant  Value=0  VectorParams1D=off
  Data Type Conversion1 : DataTypeConversion  OutDataTypeStr=double  SaturateOnIntegerOverflow=on  RndMeth=Zero
  Relational Operator2 : RelationalOperator  RndMeth=Nearest  InputSameDT=on
  Sample and Hold : dspsigops/Sample and Hold  trig=Either edge  initCond=0  latchinput=off
  Out1 : Outport
  wires:
  b1/1 -> Sample and Hold/1
  Constant5/1 -> Relational Operator2/2
  Relational Operator2/1 -> Data Type Conversion1/1
  In2/1 -> Relational Operator2/1
  Data Type Conversion1/1 -> Sample and Hold/Trigger
  Sample and Hold/1 -> Abs/1
  Abs/1 -> Out1/1

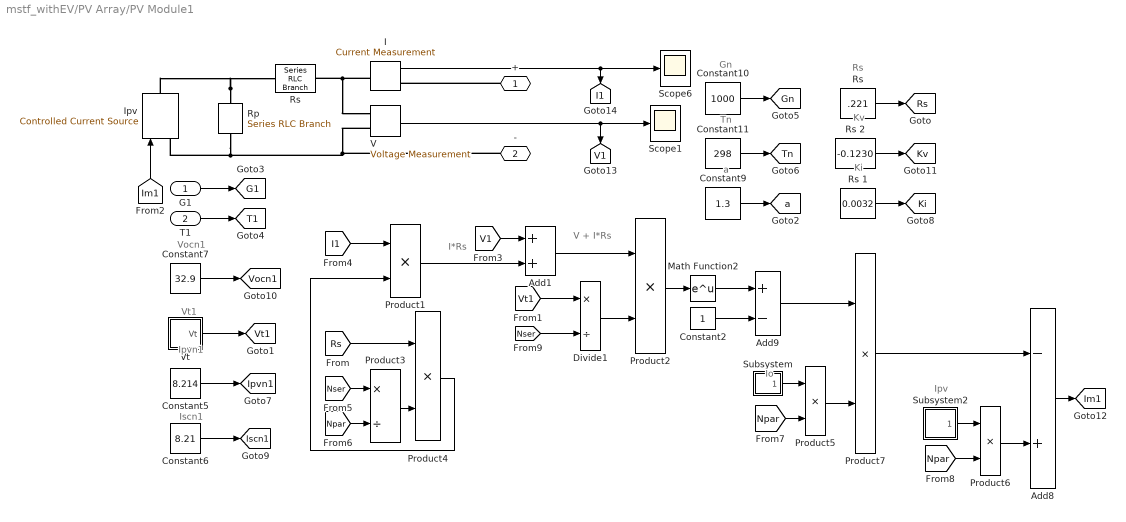
== system mstf_withEV/PV Array/PV Module1 ==
  note: Vocn1
  note: Iscn1
  note: Ipvn1
  note: I*Rs
  note: Vt1
  note: V + I*Rs
  note: Io
  note: Kv
  note: Ki
  note: Tn
  note: Gn
  note: Rs
  note: a
  note: Ipv
  G1 : Inport
  T1 : Inport  Port=2
  Add1 : Sum
  Add8 : Sum  Inputs=-+
  Add9 : Sum  Inputs=+-
  Constant10 : Constant  Value=1000
  Constant11 : Constant  Value=298
  Constant2 : Constant
  Constant5 : Constant  Value=8.214
  Constant6 : Constant  Value=8.21
  Constant7 : Constant  Value=32.9
  Constant9 : Constant  Value=1.3
  Divide1 : Product  Inputs=*/
  I : spsCurrentMeasurementLib/Current Measurement  PhasorSimulation=off  OutputType=Complex  PSBequivalent=0
  Ipv : spsControlledCurrentSourceLib/Controlled Current Source  Initialize=on  Source_Type=DC  Amplitude=0  Phase=0  Frequency=0  Measurements=None
  Math Function2 : Math  SignedPower=on  SaturateOnIntegerOverflow=on
  Product{1..2,4..7} (6 alike) : Product  RndMeth=Zero
  Product3 : Product  Inputs=*/  RndMeth=Zero
  Rp : spsSeriesRLCBranchLib/Series RLC Branch  LConnTagsString=__new0  RConnTagsString=__new0  BranchType=R  Resistance=3460.32  Inductance=1e-3  SetiL0=off  InitialCurrent=0  Capacitance=1e-6  Setx0=off  InitialVoltage=0  Measurements=None
  Rs : spsSeriesRLCBranchLib/Series RLC Branch  LConnTagsString=__new0  RConnTagsString=__new0  BranchType=R  Resistance=1.84  Inductance=1e-3  SetiL0=off  InitialCurrent=0  Capacitance=1e-6  Setx0=off  InitialVoltage=0  Measurements=None
  "Rs " : Constant  Value=.221
  Rs 1 : Constant  Value=0.0032
  Rs 2 : Constant  Value=-0.1230
  Scope1 : Scope
  Scope6 : Scope
  Subsystem : Subsystem
  Subsystem2 : Subsystem
  "V " : spsVoltageMeasurementLib/Voltage Measurement  PhasorSimulation=off  OutputType=Complex  PSBequivalent=0
  Vt : Subsystem
  + : PMIOPort  Side=Right
  - : PMIOPort  Port=2  Side=Right
  tag scope: G1=global, Gn=global, I1=global, Im1=global, Ipvn1=global, Iscn1=global, Ki=global, Kv=global, Rs=global, T1=global, Tn=global, V1=global, Vocn1=global, Vt1=global, a=global
  wires:
  "V "/1 -> Scope1/1, [V1]
  [I1] -> Product1/1
  [V1] -> Add1/1
  [Im1] -> Ipv/1
  Add8/1 -> [Im1]
  I/1 -> Scope6/1, [I1]
  Product7/1 -> Add8/1
  Add9/1 -> Product7/1
  Constant7/1 -> [Vocn1]
  Constant6/1 -> [Iscn1]
  Constant5/1 -> [Ipvn1]
  T1/1 -> [T1]
  G1/1 -> [G1]
  Vt/1(Vt) -> [Vt1]
  Constant2/1 -> Add9/2
  Math Function2/1 -> Add9/1
  Product2/1 -> Math Function2/1
  Add1/1 -> Product2/1
  Product1/1 -> Add1/2
  Rs 2/1 -> [Kv]
  Rs 1/1 -> [Ki]
  Constant11/1 -> [Tn]
  Constant10/1 -> [Gn]
  Constant9/1 -> [a]
  "Rs "/1 -> [Rs]
  [Nser] -> Product3/1
  [Npar] -> Product3/2
  Product3/1 -> Product4/2
  [Npar] -> Product6/2
  [Rs] -> Product4/1
  Product4/1 -> Product1/2
  Subsystem/1(Out1) -> Product5/1
  [Npar] -> Product5/2
  Product5/1 -> Product7/2
  Subsystem2/1(Out1) -> Product6/1
  Product6/1 -> Add8/2
  [Nser] -> Divide1/2
  [Vt1] -> Divide1/1
  Divide1/1 -> Product2/2
  connections:
  +/RConn1 -- I/RConn1
  "V "/LConn2 -- -/RConn1 -- Rp/RConn1 -- Ipv/LConn1
  Rp/LConn1 -- Ipv/RConn1 -- Rs/LConn1
  I/LConn1 -- Rs/RConn1 -- "V "/LConn1

== system mstf_withEV/Control Algorithm/Self Tuning Filter/Subsystem2 ==
  a : Inport
  a2 : Inport  Port=2
  a4 : Inport  Port=3
  Subsystem : Subsystem
  Subsystem1 : Subsystem
  Subsystem2 : Subsystem
  a1 : Outport
  a3 : Outport  Port=2
  a5 : Outport  Port=3
  wires:
  a/1 -> Subsystem/1(a)
  Subsystem/1(a1) -> a1/1
  a2/1 -> Subsystem1/1(a)
  Subsystem1/1(a1) -> a3/1
  a4/1 -> Subsystem2/1(a)
  Subsystem2/1(a1) -> a5/1

== system mstf_withEV/Control Algorithm/Subsystem2/Self Tuning Filter ==
  a : Inport
  b : Inport  Port=2
  c : Inport  Port=3
  Subsystem2 : Subsystem
  a1 : Outport
  b1 : Outport  Port=2
  c1 : Outport  Port=3
  wires:
  a/1 -> Subsystem2/1(a)
  b/1 -> Subsystem2/2(a2)
  c/1 -> Subsystem2/3(a4)
  Subsystem2/1(a1) -> a1/1
  Subsystem2/2(a3) -> b1/1
  Subsystem2/3(a5) -> c1/1

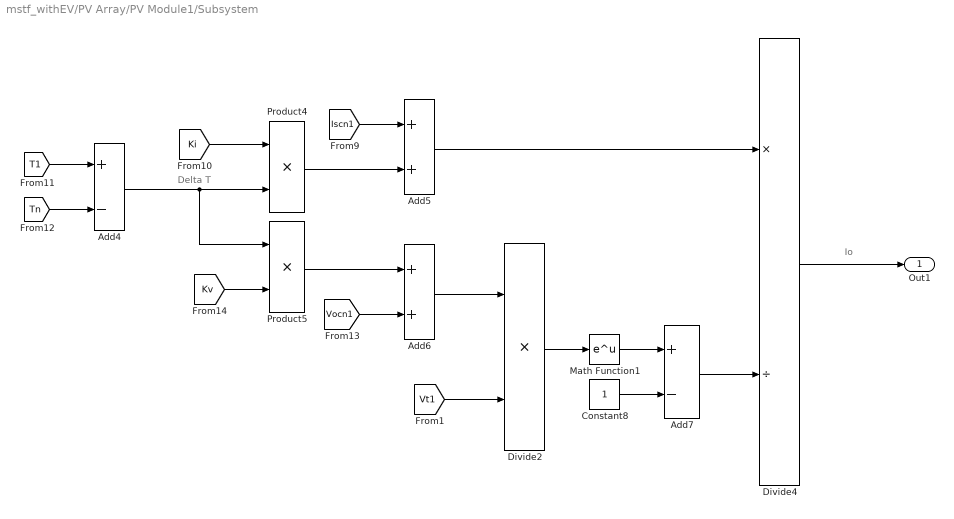
== system mstf_withEV/PV Array/PV Module1/Subsystem ==
  note: Delta T
  note: Io
  Add4 : Sum  Inputs=+-
  Add5 : Sum
  Add6 : Sum
  Add7 : Sum  Inputs=+-
  Constant8 : Constant
  Divide2 : Product  Inputs=**
  Divide4 : Product  Inputs=*/
  Math Function1 : Math  SignedPower=on  SaturateOnIntegerOverflow=on
  Product4 : Product  RndMeth=Zero
  Product5 : Product  RndMeth=Zero
  Out1 : Outport
  wires:
  [Vt1] -> Divide2/2
  Divide4/1 -> Out1/1
  Add7/1 -> Divide4/2
  Divide2/1 -> Math Function1/1
  Constant8/1 -> Add7/2
  Math Function1/1 -> Add7/1
  Add6/1 -> Divide2/1
  Product5/1 -> Add6/1
  [Kv] -> Product5/2
  [Vocn1] -> Add6/2
  [Tn] -> Add4/2
  Add5/1 -> Divide4/1
  [Iscn1] -> Add5/1
  Product4/1 -> Add5/2
  [Ki] -> Product4/1
  Add4/1 -> Product5/1, Product4/2
  [T1] -> Add4/1

== system mstf_withEV/PV Array/PV Module1/Subsystem2 ==
  note: Ipv
  note: Delta T
  Add2 : Sum  Inputs=+-
  Add3 : Sum
  Divide1 : Product  Inputs=*/
  Product2 : Product  RndMeth=Zero
  Product3 : Product  RndMeth=Zero
  Out1 : Outport
  wires:
  [G1] -> Divide1/1
  [Gn] -> Divide1/2
  Divide1/1 -> Product3/2
  [Tn] -> Add2/2
  [T1] -> Add2/1
  Add2/1 -> Product2/2
  [Ki] -> Product2/1
  Product2/1 -> Add3/2
  [Ipvn1] -> Add3/1
  Add3/1 -> Product3/1
  Product3/1 -> Out1/1

== system mstf_withEV/PV Array/PV Module1/Vt ==
  note: Ns
  note: K
  note: q
  note: a
  note: T1
  Constant1 : Constant  Value=54
  Constant3 : Constant  Value=1.3806503e-23
  Constant6 : Constant  Value=1.60217646e-19
  Divide2 : Product  Inputs=*/
  Divide3 : Product  Inputs=/*
  Divide4 : Product  Inputs=***
  Vt : Outport
  wires:
  Divide3/1 -> Divide2/1
  Divide4/1 -> Divide3/1
  [T1] -> Divide2/2
  Constant6/1 -> Divide3/2
  Constant3/1 -> Divide4/3
  Constant1/1 -> Divide4/2
  [a] -> Divide4/1
  Divide2/1 -> Vt/1

== system mstf_withEV/Control Algorithm/Self Tuning Filter/Subsystem2/Subsystem ==
  a : Inport
  Constant : Constant  Value=314
  Gain : Gain  Gain=10
  Integrator : Integrator
  Integrator1 : Integrator
  Product : Product
  Product1 : Product
  Scope : Scope
  Sum : Sum  Inputs=-+
  Sum1 : Sum  Inputs=|+-
  a1 : Outport
  wires:
  Sum/1 -> Gain/1
  a/1 -> Sum/2
  Integrator/1 -> a1/1, Sum/1, Product/1
  Gain/1 -> Sum1/1
  Integrator1/1 -> Product1/1
  Sum1/1 -> Integrator/1
  Product/1 -> Integrator1/1
  Product1/1 -> Sum1/2
  Constant/1 -> Product1/2, Product/2, Scope/1

== system mstf_withEV/Control Algorithm/Self Tuning Filter/Subsystem2/Subsystem1 ==
  a : Inport
  Constant : Constant  Value=314
  Gain : Gain  Gain=10
  Integrator : Integrator
  Integrator1 : Integrator
  Product : Product
  Product1 : Product
  Scope : Scope
  Sum : Sum  Inputs=-+
  Sum1 : Sum  Inputs=|+-
  a1 : Outport
  wires:
  Sum/1 -> Gain/1
  a/1 -> Sum/2
  Integrator/1 -> a1/1, Sum/1, Product/1
  Gain/1 -> Sum1/1
  Integrator1/1 -> Product1/1
  Sum1/1 -> Integrator/1
  Product/1 -> Integrator1/1
  Product1/1 -> Sum1/2
  Constant/1 -> Product1/2, Product/2, Scope/1

== system mstf_withEV/Control Algorithm/Self Tuning Filter/Subsystem2/Subsystem2 ==
  a : Inport
  Constant : Constant  Value=314
  Gain : Gain  Gain=10
  Integrator : Integrator
  Integrator1 : Integrator
  Product : Product
  Product1 : Product
  Scope : Scope
  Sum : Sum  Inputs=-+
  Sum1 : Sum  Inputs=|+-
  a1 : Outport
  wires:
  Sum/1 -> Gain/1
  a/1 -> Sum/2
  Integrator/1 -> a1/1, Sum/1, Product/1
  Gain/1 -> Sum1/1
  Integrator1/1 -> Product1/1
  Sum1/1 -> Integrator/1
  Product/1 -> Integrator1/1
  Product1/1 -> Sum1/2
  Constant/1 -> Product1/2, Product/2, Scope/1

== system mstf_withEV/Control Algorithm/Subsystem2/Self Tuning Filter/Subsystem2 ==
  a : Inport
  a2 : Inport  Port=2
  a4 : Inport  Port=3
  Subsystem : Subsystem
  Subsystem1 : Subsystem
  Subsystem2 : Subsystem
  a1 : Outport
  a3 : Outport  Port=2
  a5 : Outport  Port=3
  wires:
  a/1 -> Subsystem/1(a)
  Subsystem/1(a1) -> a1/1
  a2/1 -> Subsystem1/1(a)
  Subsystem1/1(a1) -> a3/1
  a4/1 -> Subsystem2/1(a)
  Subsystem2/1(a1) -> a5/1

== system mstf_withEV/Control Algorithm/Subsystem2/Self Tuning Filter/Subsystem2/Subsystem ==
  a : Inport
  Constant : Constant  Value=314
  Gain : Gain  Gain=10
  Integrator : Integrator
  Integrator1 : Integrator
  Product : Product
  Product1 : Product
  Scope : Scope
  Sum : Sum  Inputs=-+
  Sum1 : Sum  Inputs=|+-
  a1 : Outport
  wires:
  Sum/1 -> Gain/1
  a/1 -> Sum/2
  Integrator/1 -> a1/1, Sum/1, Product/1
  Gain/1 -> Sum1/1
  Integrator1/1 -> Product1/1
  Sum1/1 -> Integrator/1
  Product/1 -> Integrator1/1
  Product1/1 -> Sum1/2
  Constant/1 -> Product1/2, Product/2, Scope/1

== system mstf_withEV/Control Algorithm/Subsystem2/Self Tuning Filter/Subsystem2/Subsystem1 ==
  a : Inport
  Constant : Constant  Value=314
  Gain : Gain  Gain=10
  Integrator : Integrator
  Integrator1 : Integrator
  Product : Product
  Product1 : Product
  Scope : Scope
  Sum : Sum  Inputs=-+
  Sum1 : Sum  Inputs=|+-
  a1 : Outport
  wires:
  Sum/1 -> Gain/1
  a/1 -> Sum/2
  Integrator/1 -> a1/1, Sum/1, Product/1
  Gain/1 -> Sum1/1
  Integrator1/1 -> Product1/1
  Sum1/1 -> Integrator/1
  Product/1 -> Integrator1/1
  Product1/1 -> Sum1/2
  Constant/1 -> Product1/2, Product/2, Scope/1

== system mstf_withEV/Control Algorithm/Subsystem2/Self Tuning Filter/Subsystem2/Subsystem2 ==
  a : Inport
  Constant : Constant  Value=314
  Gain : Gain  Gain=10
  Integrator : Integrator
  Integrator1 : Integrator
  Product : Product
  Product1 : Product
  Scope : Scope
  Sum : Sum  Inputs=-+
  Sum1 : Sum  Inputs=|+-
  a1 : Outport
  wires:
  Sum/1 -> Gain/1
  a/1 -> Sum/2
  Integrator/1 -> a1/1, Sum/1, Product/1
  Gain/1 -> Sum1/1
  Integrator1/1 -> Product1/1
  Sum1/1 -> Integrator/1
  Product/1 -> Integrator1/1
  Product1/1 -> Sum1/2
  Constant/1 -> Product1/2, Product/2, Scope/1

== matlab function mstf_withEV/MPPT ==
  settings: updateMethod=DISCRETE  sampleTime=1e-4
  data: tv input; Ipvin input; Vpvin input; Ipvin1 input; Vpvin1 input; Vdcref output; Vdcrefold input
function Vdcref = fcn(tv,Ipvin,Vpvin,Ipvin1,Vpvin1,Vdcrefold)
%#codegen
delVdc=0.2;
a=10;
delVpv=Vpvin-Vpvin1;
delIpv=Ipvin-Ipvin1;
if(tv>=0.6)
if(delVpv==0)
    if(delIpv==0)
        Vdcrefnew=Vdcrefold;
    else
        if(delIpv>0)
            Vdcrefnew=Vdcrefold-(delIpv/delVpv)*a;
    else
        Vdcrefnew=Vdcrefold+(delIpv/delVpv)*a;
        end
    end
    else
        if(delIpv/delVpv==-Ipvin/Vpvin)
            Vdcrefnew=Vdcrefold;
        else
            if(delIpv/delVpv>-Ipvin/Vpvin)
                Vdcrefnew=Vdcrefold-(delIpv/delVpv)*a;
            else
                Vdcrefnew=Vdcrefold+(delIpv/delVpv)*a;
            end
        end
end
Vdcref=Vdcrefnew;
else
Vdcref=810;
end


%Vdcref=658;
